simulink model "fzjt"  (R2021a)
settings: Solver=VariableStepAuto  StartTime=0.0  StopTime=10.0  RelTol=1e-3
values from neighbouring files (symbols this model uses):
  Ts = 0.5    [Distillation_Column_model_identification.m]    (also in Distillation_Column_model_variance.m; fourvary.m = 8)
libraries: cstblocks x3, dspsrcs4 x2
settings Model: Creator=dell  LastModifiedBy=dell

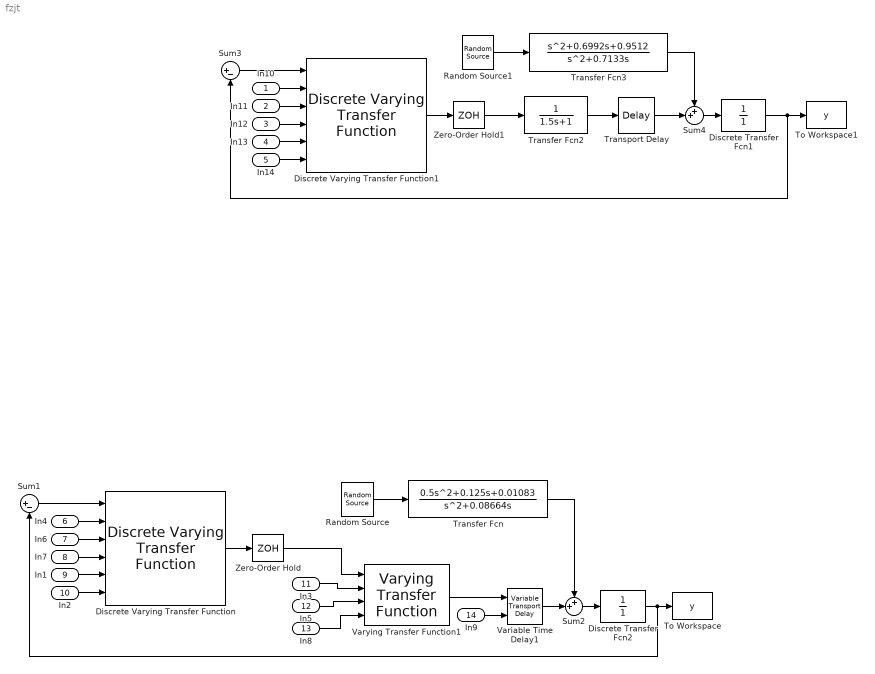
== system fzjt ==
  In10 : Inport
  In11 : Inport  Port=2
  In12 : Inport  Port=3
  In13 : Inport  Port=4
  In14 : Inport  Port=5
  In4 : Inport  Port=6
  In6 : Inport  Port=7
  In7 : Inport  Port=8
  In1 : Inport  Port=9
  In2 : Inport  Port=10
  In3 : Inport  Port=11
  In5 : Inport  Port=12
  In8 : Inport  Port=13
  In9 : Inport  Port=14
  Discrete Transfer Fcn1 : DiscreteTransferFcn  Denominator=[1]  SampleTime=Ts
      mask Display: disp('sampler')
  Discrete Transfer Fcn2 : DiscreteTransferFcn  Denominator=[1]  SampleTime=Ts
      mask Display: disp('sampler')
  Discrete Varying Transfer Function : cstblocks/Linear Parameter Varying/Discrete Varying Transfer Function  N=2  Ts=-1
      settings: SourceProductBaseCode=CT
  Discrete Varying Transfer Function1 : cstblocks/Linear Parameter Varying/Discrete Varying Transfer Function  N=2  Ts=-1
      settings: SourceProductBaseCode=CT
  Random Source : dspsrcs4/Random Source  SrcType=Gaussian  NormMethod=Ziggurat  CltLength=12  MinVal=-1  MaxVal=1  MeanVal=0  VarVal=1  RepMode=Specify seed  rawSeed=seed  IsInherit=off  SampMode=Continuous  SampTime=1  SampFrame=1  DataType=Double  OutComplex=Real  OutputFrames=off
  Random Source1 : dspsrcs4/Random Source  SrcType=Gaussian  NormMethod=Ziggurat  CltLength=12  MinVal=-1  MaxVal=1  MeanVal=0  VarVal=1  RepMode=Specify seed  rawSeed=seed  IsInherit=off  SampMode=Continuous  SampTime=1  SampFrame=1  DataType=Double  OutComplex=Real  OutputFrames=off
  Sum1 : Sum  Inputs=|+-
  Sum2 : Sum  Inputs=++|
  Sum3 : Sum  Inputs=|+-
  Sum4 : Sum  Inputs=++|
  To Workspace : ToWorkspace  VariableName=y  SampleTime=Ts
  To Workspace1 : ToWorkspace  VariableName=y  SampleTime=Ts
  Transfer Fcn : TransferFcn  Numerator=[0.5 0.125 0.01083]  Denominator=[1 0.08664 0]
  Transfer Fcn2 : TransferFcn  Denominator=[1.5 1]
  Transfer Fcn3 : TransferFcn  Numerator=[1 0.6992 0.9512]  Denominator=[1 0.7133 0]
  Transport Delay : TransportDelay  DelayTime=5
  Variable Time Delay1 : VariableTransportDelay  MaximumDelay=200
  Varying Transfer Function1 : cstblocks/Linear Parameter Varying/Varying Transfer Function  N=1
  Zero-Order Hold : ZeroOrderHold  SampleTime=Ts
  Zero-Order Hold1 : ZeroOrderHold  SampleTime=Ts
  wires:
  Varying Transfer Function1/1 -> Variable Time Delay1/1
  In5/1 -> Varying Transfer Function1/3
  In3/1 -> Varying Transfer Function1/2
  Discrete Varying Transfer Function/1 -> Zero-Order Hold/1
  Random Source/1 -> Transfer Fcn/1
  Discrete Transfer Fcn2/1 -> To Workspace/1, Sum1/2
  Transfer Fcn/1 -> Sum2/1
  In7/1 -> Discrete Varying Transfer Function/4
  In4/1 -> Discrete Varying Transfer Function/2
  In2/1 -> Discrete Varying Transfer Function/6
  In6/1 -> Discrete Varying Transfer Function/3
  In8/1 -> Varying Transfer Function1/4
  In1/1 -> Discrete Varying Transfer Function/5
  Sum2/1 -> Discrete Transfer Fcn2/1
  Variable Time Delay1/1 -> Sum2/2
  Sum1/1 -> Discrete Varying Transfer Function/1
  In9/1 -> Variable Time Delay1/2
  Zero-Order Hold/1 -> Varying Transfer Function1/1
  Sum3/1 -> Discrete Varying Transfer Function1/1
  In12/1 -> Discrete Varying Transfer Function1/4
  Sum4/1 -> Discrete Transfer Fcn1/1
  In11/1 -> Discrete Varying Transfer Function1/3
  In13/1 -> Discrete Varying Transfer Function1/5
  In14/1 -> Discrete Varying Transfer Function1/6
  Transfer Fcn3/1 -> Sum4/1
  In10/1 -> Discrete Varying Transfer Function1/2
  Discrete Transfer Fcn1/1 -> To Workspace1/1, Sum3/2
  Discrete Varying Transfer Function1/1 -> Zero-Order Hold1/1
  Random Source1/1 -> Transfer Fcn3/1
  Zero-Order Hold1/1 -> Transfer Fcn2/1
  Transfer Fcn2/1 -> Transport Delay/1
  Transport Delay/1 -> Sum4/2
